simulink model "constrained_second_link2"  (R2020b)
settings: Solver=VariableStepAuto  StartTime=0.0  StopTime=500  RelTol=1e-3
values from neighbouring files (symbols this model uses):
  b1 = 5.33518    [Linearization.m]    (also in MainScript_PID.m; calib_up_up.m; tune_parameters.m = 4.8; tune_parameters_cl.m)
  b2 = 4e-05    [Linearization.m]    (also in MainScript_PID.m; calib_up_up.m; tune_parameters.m = 5e-05; tune_parameters_cl.m = 3.7644e-05)
  c1 = 0.01    [Linearization.m]    (also in MainScript_PID.m; calib_up_up.m; tune_parameters.m = -0.04; tune_parameters_cl.m = 0.025)
  c2 = 0.07    [Linearization.m]    (also in MainScript_PID.m; calib_up_up.m; tune_parameters.m = 0.0644; tune_parameters_cl.m = 0.0644)
  g = 9.81    [Linearization.m]    (also in MainScript_PID.m; calib_up_up.m; tune_parameters.m; tune_parameters_cl.m)
  I1 = 0.01076    [Linearization.m]    (also in MainScript_PID.m; calib_up_up.m; tune_parameters.m = 0.074; tune_parameters_cl.m = 0.018544)
  I2 = 0.0001    [Linearization.m]    (also in MainScript_PID.m; calib_up_up.m; tune_parameters.m; tune_parameters_cl.m = 8.3382e-05)
  km = 39.2954    [Linearization.m]    (also in MainScript_PID.m = 42.2954; calib_up_up.m; tune_parameters.m = 50; tune_parameters_cl.m)
  l1 = 0.0897    [Linearization.m]    (also in MainScript_PID.m; calib_up_up.m; tune_parameters.m = 0.1; tune_parameters_cl.m)
  m1 = 0.2    [Linearization.m]    (also in MainScript_PID.m; calib_up_up.m; tune_parameters.m = 0.125; tune_parameters_cl.m = 0.53513)
  m2 = 0.087972    [Linearization.m]    (also in MainScript_PID.m; calib_up_up.m; tune_parameters.m = 0.0528; tune_parameters_cl.m = 0.0528)
  te = 0.01    [Linearization.m]    (also in MainScript_PID.m = 0.008; calib_up_up.m; tune_parameters.m = 0.03; tune_parameters_cl.m = 0.00258)
  theta0 = [-pi;3*pi/4]    [Compute_whitebox.m]    (also in MainScript_PID.m = [-pi;     pi/4]; calib_up_up.m = [0;-pi]; tune_parameters.m = [-pi;10*pi/12]; tune_parameters_cl.m = [-pi;-pi])
  thetadot0 = [0;0]    [MainScript_PID.m]    (also in calib_up_up.m; tune_parameters.m; tune_parameters_cl.m; tune_parameters_theta1.m)
settings Model: Creator=llaporte  LastModifiedBy=llaporte

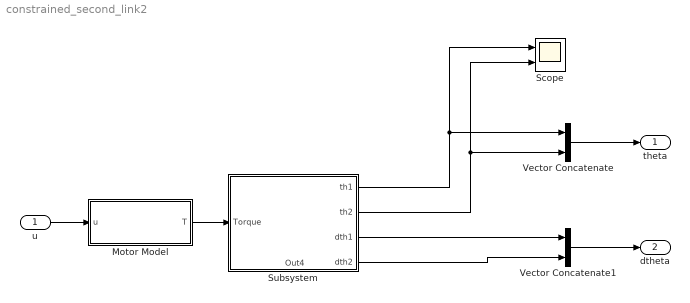
== system constrained_second_link2 ==
  u : Inport
  "Motor Model " : Subsystem
  Scope : Scope  NumInputPorts=2
  Subsystem : Subsystem
      settings: PortSchema="{\"entries\":[{\"content\":{\"sides\":[{\"content\":{\"connectorIds\":[\"In1\"]},\"type\":\"ConnectorPlacement.EquallySpacedRectSide\",\"uuid\":\"550e1cda-c923-4cd7-8fca-827ebc06ac0d\"},{\"content\":{\"connectorIds\":[\"Out1\",\"Out2\",\"Out3\",\"Out4\"],\"side\":\"RIGHT\"},\"type\":\"ConnectorPlacement.EquallySpacedRectSide\",\"uuid\":\"920df8af-3423-40a4-8eb5-84941c7c0c25\"},{\"content\":{\"connectorIds\":[],\"side\":\"TOP\"},\"type\":\"ConnectorPlacement.EquallySpacedRectSide\",\"uuid\":\"75638c39-ff1c-48c1-b3e4-9a2bdc8fca2f\"},{\"content\":{\"connectorIds\":[\"Out5\"],\"side\":\"BOTTOM\"},\"type\":\"ConnectorPlacement.EquallySpacedRectSide\",\"uuid\":\"ab57a02e-3fe6-498f-a950-7cdb8dc76560\"},{\"content\":{\"connectorIds\":[],\"side\":\"HIDDEN\"},\"type\":\"ConnectorPlacement.EquallySpacedRectSide\",\"uuid\":\"630ddbb9-257a-42a4-8f89-c3799ede61a3\"}]},\"type\":\"ConnectorPlacement.EquallySpacedConnector\",\"uuid\":\"c979b3d7-7b64-4b67-8e4c-71ddff4e7103\"}],\"packageUris\":[\"http://schema.mathworks.com/mf0/Connector/R2020b\"],\"version\":\"1.0\"}"
  Vector Concatenate : Concatenate
  Vector Concatenate1 : Concatenate
  theta : Outport
  dtheta : Outport  Port=2
  wires:
  u/1 -> "Motor Model "/1(u)
  Subsystem/2(th2) -> Vector Concatenate/2, Scope/2
  Subsystem/1(th1) -> Scope/1, Vector Concatenate/1
  Subsystem/3(dth1) -> Vector Concatenate1/1
  Subsystem/4(dth2) -> Vector Concatenate1/2
  "Motor Model "/1(T) -> Subsystem/1(Torque)
  Vector Concatenate/1 -> theta/1
  Vector Concatenate1/1 -> dtheta/1

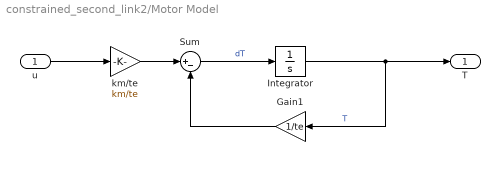
== system constrained_second_link2/Motor Model  ==
  u : Inport
  Gain1 : Gain  Gain=1/te
  Integrator : Integrator
  Sum : Sum  Inputs=|+-
  "km/te " : Gain  Gain=km/te
  T : Outport
  wires:
  "km/te "/1 -> Sum/1
  u/1 -> "km/te "/1
  Integrator/1 -> T/1, Gain1/1  "T"
  Sum/1 -> Integrator/1  "dT"
  Gain1/1 -> Sum/2

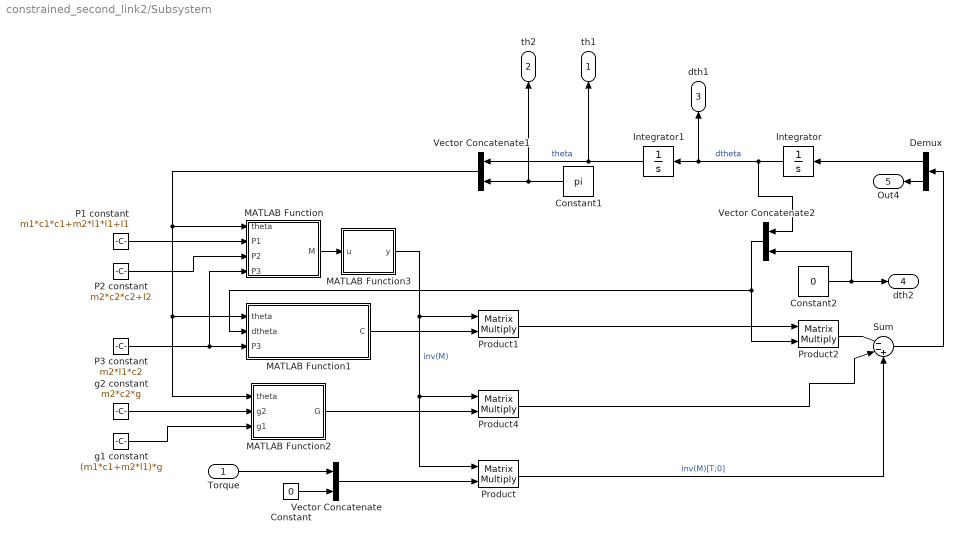
== system constrained_second_link2/Subsystem ==
  Torque : Inport
  Constant : Constant  Value=0
  Constant1 : Constant  Value=pi
  Constant2 : Constant  Value=0
  Demux : Demux  Outputs=2
  Integrator : Integrator  InitialCondition=thetadot0(1)
  Integrator1 : Integrator  InitialCondition=theta0(1)
  MATLAB Function : MATLAB Function  TreatAsAtomicUnit=on
  MATLAB Function1 : MATLAB Function  TreatAsAtomicUnit=on
  MATLAB Function2 : MATLAB Function  TreatAsAtomicUnit=on
  MATLAB Function3 : MATLAB Function  TreatAsAtomicUnit=on
  P1 constant : Constant  Value=m1*c1*c1+m2*l1*l1+I1
  P2 constant : Constant  Value=m2*c2*c2+I2
  P3 constant : Constant  Value=m2*l1*c2
  Product{,1..2,4} (4 alike) : Product  Multiplication=Matrix(*)
  Sum : Sum  Inputs=|--+
  Vector Concatenate : Concatenate
  Vector Concatenate1 : Concatenate
  Vector Concatenate2 : Concatenate
  g1 constant : Constant  Value=(m1*c1+m2*l1)*g
  g2 constant : Constant  Value=m2*c2*g
  th1 : Outport
  th2 : Outport  Port=2
  dth1 : Outport  Port=3
  dth2 : Outport  Port=4
  Out4 : Outport  Port=5
  wires:
  P2 constant/1 -> MATLAB Function/3(P2)
  Vector Concatenate1/1 -> MATLAB Function/1(theta), MATLAB Function2/1(theta), MATLAB Function1/1(theta)
  Vector Concatenate2/1 -> MATLAB Function1/2(dtheta), Product2/2
  MATLAB Function3/1(y) -> Product4/1, Product/1, Product1/1  "inv(M)"
  Integrator1/1 -> th1/1, Vector Concatenate1/1  "theta"
  Vector Concatenate/1 -> Product/2
  Constant1/1 -> th2/1, Vector Concatenate1/2
  Integrator/1 -> dth1/1, Integrator1/1, Vector Concatenate2/1  "dtheta"
  Demux/1 -> Integrator/1
  Product1/1 -> Product2/1
  Demux/2 -> Out4/1
  P3 constant/1 -> MATLAB Function/4(P3), MATLAB Function1/3(P3)
  g1 constant/1 -> MATLAB Function2/3(g1)
  Product2/1 -> Sum/1
  Constant2/1 -> dth2/1, Vector Concatenate2/2
  Sum/1 -> Demux/1
  Product/1 -> Sum/3  "inv(M)[T;0]"
  Product4/1 -> Sum/2
  MATLAB Function2/1(G) -> Product4/2
  P1 constant/1 -> MATLAB Function/2(P1)
  g2 constant/1 -> MATLAB Function2/2(g2)
  Torque/1 -> Vector Concatenate/1
  MATLAB Function1/1(C) -> Product1/2
  Constant/1 -> Vector Concatenate/2
  MATLAB Function/1(M) -> MATLAB Function3/1(u)

== matlab function constrained_second_link2/Subsystem/MATLAB Function ==
  data: theta input size=2; M output; P1 input; P2 input; P3 input
function M = M_matrix(theta,P1, P2, P3)
    M = [P1+P2+2*P3*cos(theta(2)) P2+P3*cos(theta(2));
         P2+P3*cos(theta(2))      P2];

== matlab function constrained_second_link2/Subsystem/MATLAB Function1 ==
  data: theta input; C output; dtheta input; b1 parameter; b2 parameter; P3 input
function C = C_matrix(theta, dtheta,b1,b2, P3)
C = [b1-P3*dtheta(2)*sin(theta(2))  -P3*(dtheta(1)+dtheta(2))*sin(theta(2));
     P3*dtheta(1)*sin(theta(2))     b2];

== matlab function constrained_second_link2/Subsystem/MATLAB Function2 ==
  data: theta input; G output; g2 input; g1 input
function G = G_matrix(theta,g2, g1)
G = [-g1*sin(theta(1))-g2*sin(theta(1)+theta(2));
     -g2*sin(theta(1)+theta(2))];

== matlab function constrained_second_link2/Subsystem/MATLAB Function3 ==
  data: u input; y output
function y = inverse(u)
y = inv(u);
